simulink model "gear_logic"  (R2021a)
settings: Solver=FixedStepAuto  StartTime=0.0  StopTime=30  FixedStep=0.01  RelTol=1e-3  EnableMultiTasking=on
model workspace (MAT data in the model file):
  Var = 0
  downtab = [0  5  20  35; 0  5  20  35; 0  5  25  40; 0  5  30  50; 0  30  50  80; 0  30  50  80]
  downth = [0; 5; 40; 50; 90; 100]
  uptab = [10  30  50  1000000; 10  30  50  1000000; 15  30  50  1000000; 23  41  60  1000000; 40  70  100  1000000; 40  70  100  1000000]
  upth = [0; 25; 35; 50; 90; 100]
settings Model: SILPILModeSetting=veronly  ExtModeTrigDuration=10  Creator=sgirardi  LastModifiedBy=sgirardi
settings OptimizationCC: DefaultParameterBehavior=Inlined  EnhancedBackFolding=on  PassReuseOutputArgsAs=Individual arguments  ZeroExternalMemoryAtStartup=off  ZeroInternalMemoryAtStartup=off  MaxStackSize=64  OptimizeBlockOrder=speed  DifferentSizesBufferReuse=on  OptimizationCustomize=off  EfficientTunableParamExpr=on
settings DebuggingCC: ParameterTunabilityLossMsg=error
settings HardwareCC: ProdBitPerPointer=32  ProdBitPerSizeT=32  ProdBitPerPtrDiffT=32  ProdLargestAtomicInteger=Long  ProdLargestAtomicFloat=Double  ProdWordSize=32  ProdHWDeviceType=ARM Compatible->ARM Cortex
settings SFSimCC: MATLABDynamicMemAlloc=off
settings RTWCC: SystemTargetFile=ert.tlc  TemplateMakefile=ert_default_tmf  Toolchain=GNU Tools for ARM Embedded Processors
settings CodeAppCC: ForceParamTrailComments=on  IgnoreCustomStorageClasses=off  OperatorAnnotations=on  SimulinkDataObjDesc=on  SFDataObjDesc=on  InsertBlockDesc=on
settings ERTTargetCC: TargetLangStandard=C99 (ISO)  SupportContinuousTime=on  ExtModeTransport=3  ExtModeStaticAlloc=on  ExtModeStaticAllocSize=2000  ExtModeMexFile=ext_xcp  ExtModeIntrfLevel=Level2 - Open  RootIOFormat=Structure reference  ERTCustomFileTemplate=example_file_process.tlc

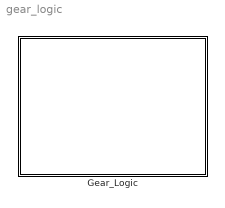
== system gear_logic ==
  Gear_Logic : Stateflow chart  TreatAsAtomicUnit=on

== stateflow chart gear_logic/Gear_Logic ==
  state gear_state [parallel]
    %on SlowDown: delta = -1;
    %on Cruise: delta = 0;
    %on SpeedUp: delta = 1;
    during:
    speed = max(0,min(speed+delta,100));
    settings: executionOrder=1
    state first
      entry:
      gear=1;
    state second
      entry:
      gear=2;
    state third
      entry:
      gear=3;
    state fourth
      entry:
      gear=4;
    (default) -> first
    first -> second : UP
    second -> third [order 1] : UP
    third -> fourth [order 1] : UP
    second -> first [order 2] : DOWN
    third -> second [order 2] : DOWN
    fourth -> third : DOWN
  state selection_state [parallel]
    during:
    computeThresholds();
    settings: executionOrder=2
    state steady_state
    state downshifting
    state upshifting
    (default) -> steady_state
    steady_state -> downshifting [order 2] : [speed < down_th]
    steady_state -> upshifting [order 1] : [speed > up_th]
    downshifting -> steady_state [order 2] : after(0.1, sec)
        | [speed <= down_th]
        | {send(DOWN, gear_state);}
    downshifting -> steady_state [order 1] : [speed > down_th]
    upshifting -> steady_state [order 2] : after(0.1, sec)
        | [speed >= up_th]
        | {send(UP,gear_state);}
    upshifting -> steady_state [order 1] : [speed < up_th]
  data: down_th local =0; up_th local =0; delta local =0.1; speed local =0; gear local =1
  events: UP local FUNCTION_CALL_EVENT; DOWN local FUNCTION_CALL_EVENT; SlowDown local RISING_EDGE_EVENT; Cruise local FUNCTION_CALL_EVENT; SpeedUp local RISING_EDGE_EVENT
  function computeThresholds:
    | function computeThresholds
    |     
    |     % turn gear light on and set tachometer coefficients
    |     switch gear
    |         case 1
    |             down_th = 0;
    |             up_th = 10;
    |             rev = interp1([0 10],[0.5 6.5],speed,'pchip','extrap');
    |         case 2
    |             rev = interp1([5 10 30],[0.5 1 6.5],speed,'pchip','extrap');
    |             down_th = 5;
    |             up_th = 30;
    |         case 3
    |             rev = interp1([25 30 50],[0.5 1 6.5],speed,'pchip','extrap');
    |             down_th = 25;
    |             up_th = 50;
    |         case 4
    |             rev = interp1([40 50 100],[0.5 1 7],speed,'pchip','extrap');
    |             down_th = 40;
    |             up_th = 100;
    |     end
    | end
